simulink model "MUL_NFB_NON_LIN"  (R2021a)
settings: Solver=VariableStepAuto  StartTime=0.0  StopTime=120  RelTol=1e-3
model workspace (MATLAB code in the model file):
  | Kia=4;
  | Kac=32;
  | Kba=10;
  | Fb=2;
  | Kcb=20;
  | Fc=6;
  | Kdc=3;
  | Kde=6;
  | Keb=6;
  | Ked=8;
  | In=0.3
  | x_star=[0.0857; 0.3000; 0.4000; 0.4500; 0.3333];
settings Model: Creator=priya  LastModifiedBy=Priyan_PC
settings SolverCC: AlgebraicLoopSolver=TrustRegion
settings DebuggingCC: SFMachineParentedDataDiag=warning

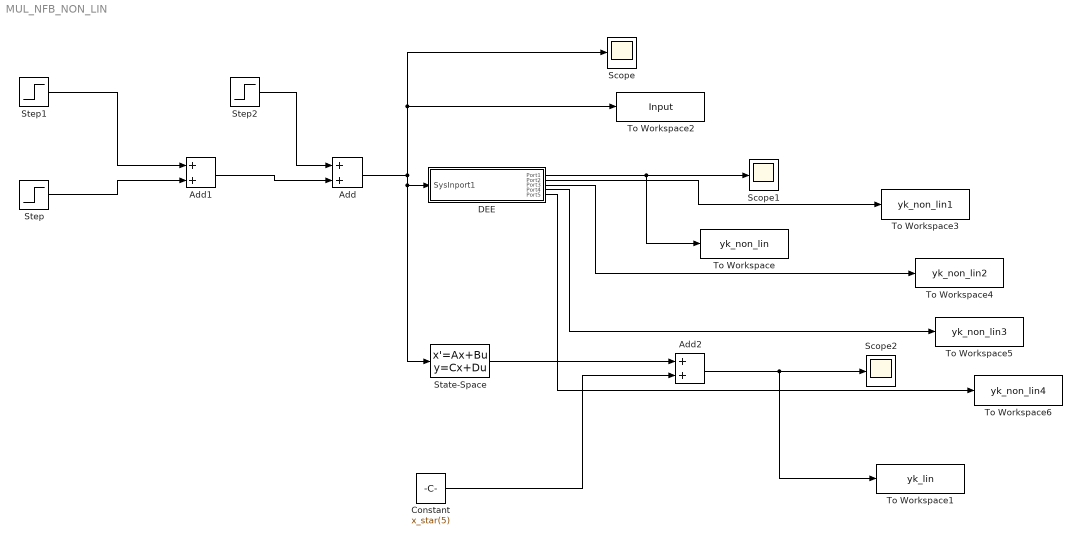
== system MUL_NFB_NON_LIN ==
  Add : Sum
  Add1 : Sum
  Add2 : Sum
  Constant : Constant  Value=x_star(5)
  DEE : Subsystem  mask(Differential Equation Editor (DEE)){}
      settings: OpenFcn=diffeqed
      mask Display: disp('Differential Equation\n Editor')
  Scope : Scope
  Scope1 : Scope
  Scope2 : Scope
  State-Space : StateSpace  A=[-12.8 0 -2.7424 0 0;7 -2.8570 0 0 0;0 20 0 0 0;0 3 0 -1.998 -2.7;0 4.0002 0 -2.6664 -5.4]  B=[3.6572;0;0;0;0]  C=[0 0 0 0 1]  D=0  InitialCondition=0
  Step : Step  Time=50  After=200  SampleTime=0
  Step1 : Step  Time=0  Before=0.3  After=50  SampleTime=0
  Step2 : Step  Time=100  After=250  SampleTime=0
  To Workspace : ToWorkspace  VariableName=yk_non_lin  SampleTime=-1
  To Workspace1 : ToWorkspace  VariableName=yk_lin  SampleTime=-1
  To Workspace2 : ToWorkspace  VariableName=Input  SampleTime=-1
  To Workspace3 : ToWorkspace  VariableName=yk_non_lin1  SampleTime=-1
  To Workspace4 : ToWorkspace  VariableName=yk_non_lin2  SampleTime=-1
  To Workspace5 : ToWorkspace  VariableName=yk_non_lin3  SampleTime=-1
  To Workspace6 : ToWorkspace  VariableName=yk_non_lin4  SampleTime=-1
  wires:
  Step1/1 -> Add1/1
  Step/1 -> Add1/2
  Add1/1 -> Add/2
  Step2/1 -> Add/1
  Add/1 -> State-Space/1, DEE/1(SysInport1), To Workspace2/1, Scope/1
  DEE/1(Port1) -> To Workspace/1, Scope1/1
  State-Space/1 -> Add2/1
  Constant/1 -> Add2/2
  Add2/1 -> To Workspace1/1, Scope2/1
  DEE/2(Port2) -> To Workspace3/1
  DEE/3(Port3) -> To Workspace4/1
  DEE/4(Port4) -> To Workspace5/1
  DEE/5(Port5) -> To Workspace6/1

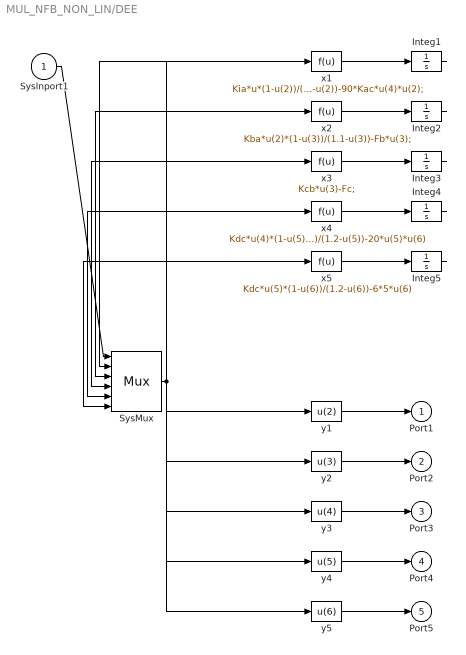
== system MUL_NFB_NON_LIN/DEE ==
  SysInport1 : Inport
  Integ1 : Integrator  InitialCondition=x_star(1)
  Integ2 : Integrator  InitialCondition=x_star(2)
  Integ3 : Integrator  InitialCondition=x_star(3)
  Integ4 : Integrator  InitialCondition=x_star(4)
  Integ5 : Integrator  InitialCondition=x_star(5)
  SysMux : Mux  Inputs=6
  x1 : Fcn  Expr=Kia*u*(1-u(2))/(1.2-u(2))-90*Kac*u(4)*u(2);
  x2 : Fcn  Expr=Kba*u(2)*(1-u(3))/(1.1-u(3))-Fb*u(3);
  x3 : Fcn  Expr=Kcb*u(3)-Fc;
  x4 : Fcn  Expr=Kdc*u(4)*(1-u(5))/(1.2-u(5))-20*u(5)*u(6)
  x5 : Fcn  Expr=Kdc*u(5)*(1-u(6))/(1.2-u(6))-6*5*u(6)
  y1 : Fcn  Expr=u(2)
  y2 : Fcn  Expr=u(3)
  y3 : Fcn  Expr=u(4)
  y4 : Fcn  Expr=u(5)
  y5 : Fcn  Expr=u(6)
  Port1 : Outport
  Port2 : Outport  Port=2
  Port3 : Outport  Port=3
  Port4 : Outport  Port=4
  Port5 : Outport  Port=5
  wires:
  SysInport1/1 -> SysMux/1
  SysMux/1 -> x1/1, x2/1, x3/1, x4/1, x5/1, y1/1, y2/1, y3/1, y4/1, y5/1
  x1/1 -> Integ1/1
  Integ1/1 -> SysMux/2
  x2/1 -> Integ2/1
  Integ2/1 -> SysMux/3
  x3/1 -> Integ3/1
  Integ3/1 -> SysMux/4
  x4/1 -> Integ4/1
  Integ4/1 -> SysMux/5
  x5/1 -> Integ5/1
  Integ5/1 -> SysMux/6
  y1/1 -> Port1/1
  y2/1 -> Port2/1
  y3/1 -> Port3/1
  y4/1 -> Port4/1
  y5/1 -> Port5/1
